simulink model "respuesta_sistema1"  (R2024a)
settings: Solver=VariableStepAuto  StartTime=0.0  StopTime=20  RelTol=1e-3

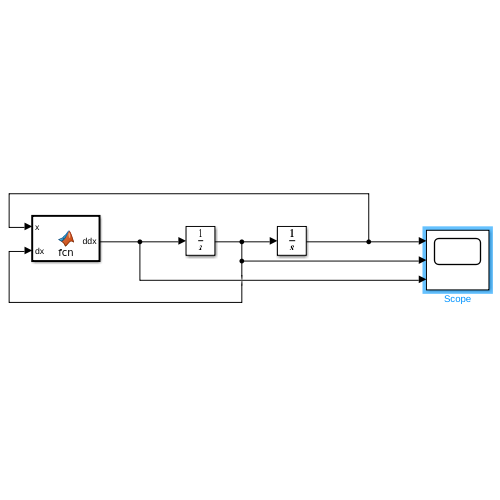
[thumbnail: Simulink's stored preview of the top-level diagram]
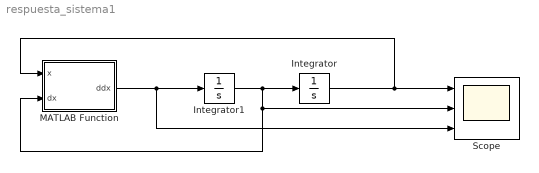
== system respuesta_sistema1 ==
  Integrator : Integrator
  Integrator1 : Integrator  InitialCondition=5
  MATLAB Function : MATLAB Function  TreatAsAtomicUnit=on
  Scope : Scope  NumInputPorts=3
  wires:
  MATLAB Function/1(ddx) -> Scope/3, Integrator1/1
  Integrator/1 -> MATLAB Function/1(x), Scope/1
  Integrator1/1 -> Scope/2, MATLAB Function/2(dx), Integrator/1

== matlab function respuesta_sistema1/MATLAB Function ==
  data: x input; ddx output; dx input
function ddx = fcn(x,dx)
k=0.01;
m=0.75;
L=0.36;
g=9.8;
tau=0;
a=L/2;
J=(4/3)*m*a*a;

ddx = (tau-((m*g*a)*cos(x))-(k*dx))/J
